simulink model "AttitudeOnly"  (R2024b)
settings: Solver=VariableStepAuto  StartTime=0.0  StopTime=10.0  FixedStep=0.00001  RelTol=1e-3
undefined symbols (not defined in the file): d, DiscIntNeverNeededParam, g, I, k_q, k_t, m, rad, s, Ts_PID_attitude, Ts_PID_position
libraries: simulink_extras x10, simulink x6, aerolibconvert2 x4, aerolibutil x2, shared6dof x1, matrix_library x1, sharedutil x1
settings Model: Creator=User  LastModifiedBy=User

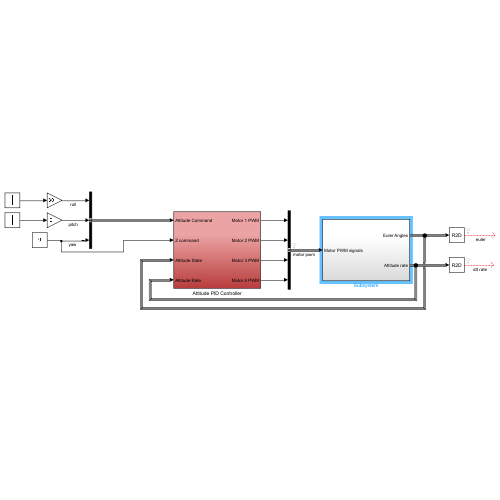
[thumbnail: Simulink's stored preview of the top-level diagram]
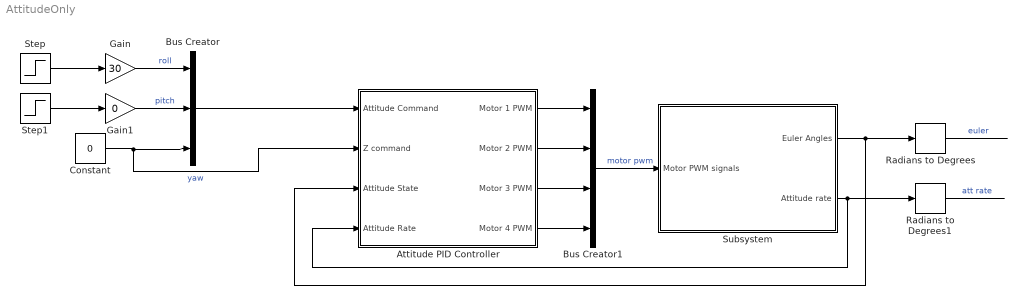
== system AttitudeOnly ==
  Attitude PID Controller : Subsystem
  Bus Creator : BusCreator  Inputs=3
  Bus Creator1 : BusCreator  Inputs=4
  Constant : Constant  Value=0
  Gain : Gain  Gain=30
  Gain1 : Gain  Gain=0
  Radians to Degrees : simulink_extras/Transformations/Radians to Degrees
  Radians to Degrees1 : simulink_extras/Transformations/Radians to Degrees
  Step : Step  Time=2  SampleTime=0
  Step1 : Step  Time=2  SampleTime=0
  Subsystem : Subsystem
  wires:
  Attitude PID Controller/2(Motor 2 PWM) -> Bus Creator1/2
  Attitude PID Controller/1(Motor 1 PWM) -> Bus Creator1/1
  Attitude PID Controller/3(Motor 3 PWM) -> Bus Creator1/3
  Attitude PID Controller/4(Motor 4 PWM) -> Bus Creator1/4
  Bus Creator1/1 -> Subsystem/1(Motor PWM signals)  "motor pwm"
  Bus Creator/1 -> Attitude PID Controller/1(Attitude Command)
  Step1/1 -> Gain1/1
  Constant/1 -> Bus Creator/3, Attitude PID Controller/2(Z command)  "yaw"
  Step/1 -> Gain/1
  Gain/1 -> Bus Creator/1  "roll"
  Gain1/1 -> Bus Creator/2  "pitch"
  Subsystem/1(Euler Angles) -> Radians to Degrees/1, Attitude PID Controller/3(Attitude State)
  Subsystem/2(Attitude rate) -> Radians to Degrees1/1, Attitude PID Controller/4(Attitude Rate)
  Radians to Degrees/1 -> ?  "euler"
  Radians to Degrees1/1 -> ?  "att rate"

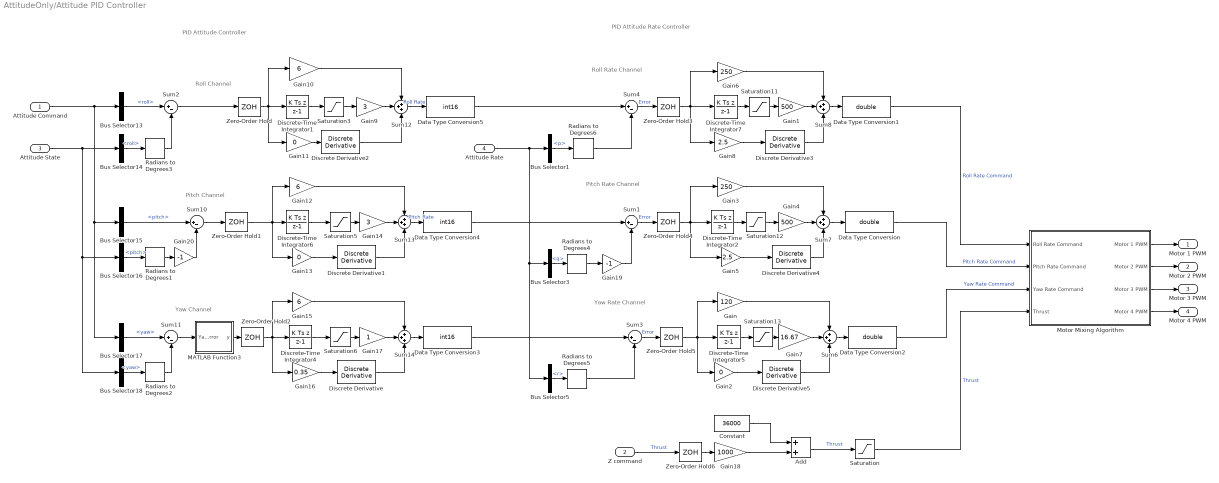
== system AttitudeOnly/Attitude PID Controller ==
  note: Yaw Rate Channel
  note: Pitch Rate Channel
  note: Roll Rate Channel
  note: Yaw Channel
  note: Pitch Channel
  note: PID Attitude Rate Controller
  note: PID Attitude Controller
  note: Roll Channel
  Attitude Command : Inport
  Z command : Inport  Port=2
  Attitude State : Inport  Port=3
  Attitude Rate : Inport  Port=4
  Add : Sum
  Bus Selector1 : BusSelector  OutputSignals=p
  Bus Selector13 : BusSelector  OutputSignals=roll
  Bus Selector14 : BusSelector  OutputSignals=roll
  Bus Selector15 : BusSelector  OutputSignals=pitch
  Bus Selector16 : BusSelector  OutputSignals=pitch
  Bus Selector17 : BusSelector  OutputSignals=yaw
  Bus Selector18 : BusSelector  OutputSignals=yaw
  Bus Selector3 : BusSelector  OutputSignals=q
  Bus Selector5 : BusSelector  OutputSignals=r
  Constant : Constant  Value=36000
  Data Type Conversion : DataTypeConversion  OutDataTypeStr=double  RndMeth=Floor
  Data Type Conversion1 : DataTypeConversion  OutDataTypeStr=double  RndMeth=Floor
  Data Type Conversion2 : DataTypeConversion  OutDataTypeStr=double  RndMeth=Floor
  Data Type Conversion3 : DataTypeConversion  OutDataTypeStr=int16  RndMeth=Floor
  Data Type Conversion4 : DataTypeConversion  OutDataTypeStr=int16  RndMeth=Floor
  Data Type Conversion5 : DataTypeConversion  OutDataTypeStr=int16  RndMeth=Floor
  Discrete Derivative{,1..5} (6 alike) : simulink/Discrete/Discrete Derivative  gainval=1.0  ICPrevScaledInput=0.0  OutMin=[]  OutMax=[]  OutDataType=fixdt(1, 16)  OutScaling=2^-10  DoSatur=off
  Discrete-Time Integrator{1..2,4..7} (6 alike) : DiscreteIntegrator  IntegratorMethod=Integration: Backward Euler  SampleTime=-1  ICPrevOutput=DiscIntNeverNeededParam  ICPrevScaledInput=DiscIntNeverNeededParam
  Gain : Gain  Gain=120
  Gain1 : Gain  Gain=500
  Gain10 : Gain  Gain=6
  Gain11 : Gain  Gain=0
  Gain12 : Gain  Gain=6
  Gain13 : Gain  Gain=0
  Gain14 : Gain  Gain=3
  Gain15 : Gain  Gain=6
  Gain16 : Gain  Gain=0.35
  Gain17 : Gain
  Gain18 : Gain  Gain=1000
  Gain19 : Gain  Gain=-1
  Gain2 : Gain  Gain=0
  Gain20 : Gain  Gain=-1
  Gain3 : Gain  Gain=250
  Gain4 : Gain  Gain=500
  Gain5 : Gain  Gain=2.5
  Gain6 : Gain  Gain=250
  Gain7 : Gain  Gain=16.67
  Gain8 : Gain  Gain=2.5
  Gain9 : Gain  Gain=3
  MATLAB Function3 : MATLAB Function  TreatAsAtomicUnit=on
  Motor Mixing Algorithm : Subsystem
  Radians to Degrees{1..6} (6 alike) : simulink_extras/Transformations/Radians to Degrees
  Saturation : Saturate  UpperLimit=65535  LowerLimit=20000
  Saturation11 : Saturate  UpperLimit=33.3  LowerLimit=-33.3
  Saturation12 : Saturate  UpperLimit=33.3  LowerLimit=-33.3
  Saturation13 : Saturate  UpperLimit=166.7  LowerLimit=-166.7
  Saturation3 : Saturate  UpperLimit=20  LowerLimit=-20
  Saturation5 : Saturate  UpperLimit=20  LowerLimit=-20
  Saturation6 : Saturate  UpperLimit=360  LowerLimit=-360
  Sum{1..4,10..11} (6 alike) : Sum  Inputs=|+-
  Sum{6..8,12..14} (6 alike) : Sum  Inputs=+++
  Zero-Order Hold{,1..5} (6 alike) : ZeroOrderHold  SampleTime=Ts_PID_attitude
  Zero-Order Hold6 : ZeroOrderHold  SampleTime=Ts_PID_position
  Motor 1 PWM : Outport
  Motor 2 PWM : Outport  Port=2
  Motor 3 PWM : Outport  Port=3
  Motor 4 PWM : Outport  Port=4
  wires:
  Constant/1 -> Add/1
  Add/1 -> Saturation/1  "Thrust"
  Bus Selector17/1 -> Sum11/1  "<yaw>"
  Motor Mixing Algorithm/4(Motor 4 PWM) -> Motor 4 PWM/1
  Motor Mixing Algorithm/3(Motor 3 PWM) -> Motor 3 PWM/1
  Motor Mixing Algorithm/2(Motor 2 PWM) -> Motor 2 PWM/1
  Motor Mixing Algorithm/1(Motor 1 PWM) -> Motor 1 PWM/1
  Sum13/1 -> Data Type Conversion4/1  "Pitch Rate"
  Sum12/1 -> Data Type Conversion5/1  "Roll Rate"
  Sum11/1 -> MATLAB Function3/1(YawError)
  Zero-Order Hold2/1 -> Discrete-Time Integrator4/1, Gain16/1, Gain15/1
  Radians to Degrees2/1 -> Sum11/2
  Saturation6/1 -> Gain17/1
  Saturation5/1 -> Gain14/1
  Saturation3/1 -> Gain9/1
  Discrete-Time Integrator4/1 -> Saturation6/1
  Discrete-Time Integrator6/1 -> Saturation5/1
  Discrete-Time Integrator1/1 -> Saturation3/1
  Saturation13/1 -> Gain7/1
  Saturation12/1 -> Gain4/1
  Saturation11/1 -> Gain1/1
  Gain16/1 -> Discrete Derivative/1
  Gain15/1 -> Sum14/1
  Gain12/1 -> Sum13/1
  Sum10/1 -> Zero-Order Hold1/1
  Gain10/1 -> Sum12/1
  Gain11/1 -> Discrete Derivative2/1
  Sum2/1 -> Zero-Order Hold/1
  Bus Selector18/1 -> Radians to Degrees2/1  "<yaw>"
  Bus Selector16/1 -> Radians to Degrees1/1  "<pitch>"
  Bus Selector14/1 -> Radians to Degrees3/1  "<roll>"
  Attitude Command/1 -> Bus Selector17/1, Bus Selector15/1, Bus Selector13/1
  Discrete-Time Integrator5/1 -> Saturation13/1
  Discrete-Time Integrator2/1 -> Saturation12/1
  Discrete-Time Integrator7/1 -> Saturation11/1
  Sum3/1 -> Zero-Order Hold5/1  "Error"
  Gain5/1 -> Discrete Derivative4/1
  Sum6/1 -> Data Type Conversion2/1
  Sum7/1 -> Data Type Conversion/1
  Sum8/1 -> Data Type Conversion1/1
  Sum4/1 -> Zero-Order Hold3/1  "Error"
  Gain6/1 -> Sum8/1
  Sum1/1 -> Zero-Order Hold4/1  "Error"
  Gain3/1 -> Sum7/1
  Gain/1 -> Sum6/1
  Attitude Rate/1 -> Bus Selector5/1, Bus Selector3/1, Bus Selector1/1
  Bus Selector5/1 -> Radians to Degrees5/1  "<r>"
  Bus Selector3/1 -> Radians to Degrees4/1  "<q>"
  Bus Selector1/1 -> Radians to Degrees6/1  "<p>"
  Gain18/1 -> Add/2
  Z command/1 -> Zero-Order Hold6/1  "Thrust"
  Attitude State/1 -> Bus Selector14/1, Bus Selector16/1, Bus Selector18/1
  Saturation/1 -> Motor Mixing Algorithm/4(Thrust)  "Thrust"
  Zero-Order Hold/1 -> Gain10/1, Discrete-Time Integrator1/1, Gain11/1
  Zero-Order Hold1/1 -> Discrete-Time Integrator6/1, Gain12/1, Gain13/1
  MATLAB Function3/1(y) -> Zero-Order Hold2/1
  Zero-Order Hold4/1 -> Discrete-Time Integrator2/1, Gain3/1, Gain5/1
  Zero-Order Hold5/1 -> Discrete-Time Integrator5/1, Gain2/1, Gain/1
  Zero-Order Hold6/1 -> Gain18/1
  Gain2/1 -> Discrete Derivative5/1
  Data Type Conversion4/1 -> Sum1/1
  Data Type Conversion1/1 -> Motor Mixing Algorithm/1(Roll Rate Command)  "Roll Rate Command"
  Data Type Conversion/1 -> Motor Mixing Algorithm/2(Pitch Rate Command)  "Pitch Rate Command"
  Data Type Conversion2/1 -> Motor Mixing Algorithm/3(Yaw Rate Command)  "Yaw Rate Command"
  Gain13/1 -> Discrete Derivative1/1
  Zero-Order Hold3/1 -> Discrete-Time Integrator7/1, Gain6/1, Gain8/1
  Gain8/1 -> Discrete Derivative3/1
  Gain4/1 -> Sum7/2
  Gain9/1 -> Sum12/2
  Gain17/1 -> Sum14/2
  Gain1/1 -> Sum8/2
  Gain14/1 -> Sum13/2
  Gain7/1 -> Sum6/2
  Bus Selector13/1 -> Sum2/1  "<roll>"
  Data Type Conversion5/1 -> Sum4/1
  Bus Selector15/1 -> Sum10/1  "<pitch>"
  Discrete Derivative3/1 -> Sum8/3
  Discrete Derivative4/1 -> Sum7/3
  Discrete Derivative/1 -> Sum14/3
  Discrete Derivative1/1 -> Sum13/3
  Discrete Derivative2/1 -> Sum12/3
  Sum14/1 -> Data Type Conversion3/1
  Data Type Conversion3/1 -> Sum3/1
  Discrete Derivative5/1 -> Sum6/3
  Radians to Degrees3/1 -> Sum2/2
  Radians to Degrees1/1 -> Gain20/1
  Gain20/1 -> Sum10/2
  Gain19/1 -> Sum1/2
  Radians to Degrees6/1 -> Sum4/2
  Radians to Degrees4/1 -> Gain19/1
  Radians to Degrees5/1 -> Sum3/2

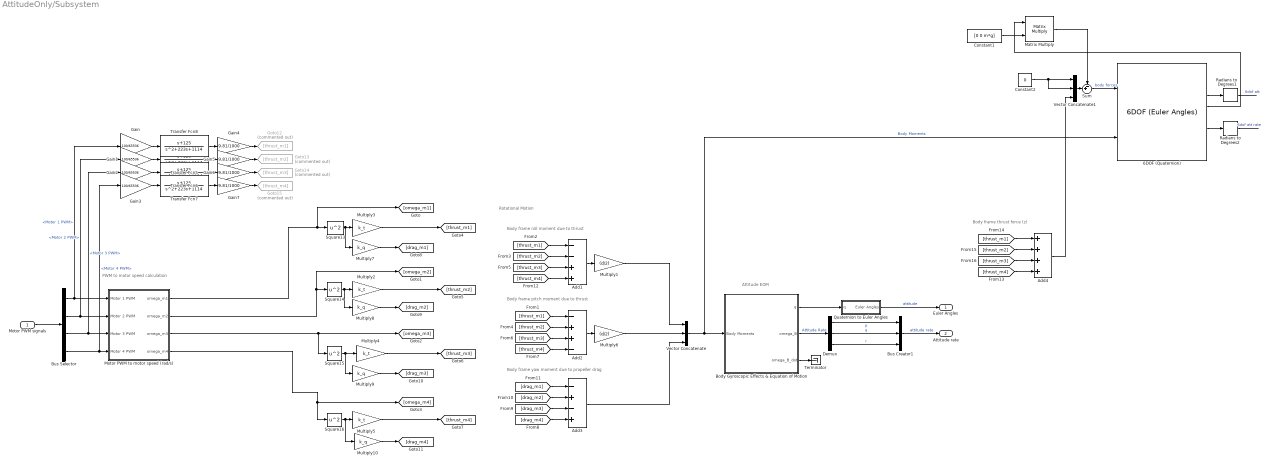
== system AttitudeOnly/Subsystem ==
  note: Body frame pitch moment due to thrust
  note: PWM to motor
      | speed calculation
  note: Rotational Motion
  note: Body frame roll moment due to thrust
  note: Attitude EOM
  note: Body frame yaw moment due to propeller drag
  note: Body frame thrust force (z)
  Motor PWM signals : Inport
  6DOF (Quaternion) : shared6dof/6DOF (Euler Angles)  units=Metric (MKS)  mtype=Fixed  rep=Quaternion  xme_0=[0 0 0.5]  Vm_0=[0 0 0]  eul_0=[0 0 0]  pm_0=[0 0 0]  mass_0=m  mass_e=0.5  mass_f=2.0  inertia=I  inertia_e=eye(3)  inertia_f=2*eye(3)  k_quat=1.0  vre_flag=on  abi_flag=off  aMode=0  xme_statename=''  Vm_statename=''  eul_statename=''  quat_statename=''  pm_statename=''  mass_statename=''
      settings: LibrarySourceBlock=aerolib6dof2/6DOF (Quaternion)
  Add1 : Sum  Inputs=--++
  Add2 : Sum  Inputs=-++-
  Add3 : Sum  Inputs=-+-+
  Add4 : Sum  Inputs=++++
  Body Gyroscopic Effects & Equation of Motion : Subsystem
  Bus Creator1 : BusCreator  Inputs=3
  Bus Selector : BusSelector  OutputSignals=Motor 1 PWM,Motor 2 PWM,Motor 3 PWM,Motor 4 PWM
  Constant1 : Constant  Value=[0 0 m*g]
  Constant2 : Constant  Value=0
  Demux : Demux  Outputs=3
  Gain{,1..3} (4 alike) : Gain  Gain=100/65536
  Gain{4..7} (4 alike) : Gain  Gain=9.81/1000
  Goto12 : Goto  Commented=on  GotoTag=thrust_m1
  Goto13 : Goto  Commented=on  GotoTag=thrust_m2
  Goto14 : Goto  Commented=on  GotoTag=thrust_m3
  Goto15 : Goto  Commented=on  GotoTag=thrust_m4
  Matrix Multiply : Product  Multiplication=Matrix(*)
  Motor PWM to motor speed (rad/s) : Subsystem
  Multiply1 : Gain  Gain=(d/2)
  Multiply{7..10} (4 alike) : Gain  Gain=k_q
  Multiply{2..5} (4 alike) : Gain  Gain=k_t
  Multiply6 : Gain  Gain=(d/2)
  Quaternion to Euler Angles : Subsystem
  Radians to Degrees1 : simulink_extras/Transformations/Radians to Degrees
  Radians to Degrees2 : simulink_extras/Transformations/Radians to Degrees
  Square{13..16} (4 alike) : Math  Operator=square
  Sum : Sum  Inputs=-+|
  Terminator : Terminator
  Transfer Fcn{5..8} (4 alike) : TransferFcn  Numerator=[1 125]  Denominator=[1 223 1114]
  Vector Concatenate : Concatenate  NumInputs=3
  Vector Concatenate1 : Concatenate  NumInputs=3
  Euler Angles : Outport
  Attitude rate : Outport  Port=2
  wires:
  Multiply7/1 -> [drag_m1]
  [thrust_m3] -> Add1/3
  [thrust_m4] -> Add2/4
  Square13/1 -> Multiply3/1, Multiply7/1
  [drag_m4] -> Add3/4
  Body Gyroscopic Effects & Equation of Motion/3(omega_B_dot) -> Terminator/1
  Bus Selector/4 -> Gain3/1, Motor PWM to motor speed (rad/s)/4(Motor 4 PWM)  "<Motor 4 PWM>"
  Multiply4/1 -> [thrust_m3]
  [thrust_m2] -> Add2/2
  Add2/1 -> Multiply6/1
  [thrust_m2] -> Add1/2
  Motor PWM signals/1 -> Bus Selector/1
  Motor PWM to motor speed (rad/s)/3(omega_m3) -> [omega_m3], Square15/1
  Square16/1 -> Multiply10/1, Multiply5/1
  Multiply8/1 -> [drag_m2]
  [drag_m1] -> Add3/1
  [thrust_m1] -> Add2/1
  Multiply1/1 -> Vector Concatenate/1
  Bus Selector/1 -> Gain/1, Motor PWM to motor speed (rad/s)/1(Motor 1 PWM)  "<Motor 1 PWM>"
  Multiply3/1 -> [thrust_m1]
  Multiply10/1 -> [drag_m4]
  Bus Selector/2 -> Gain1/1, Motor PWM to motor speed (rad/s)/2(Motor 2 PWM)  "<Motor 2 PWM>"
  Add3/1 -> Vector Concatenate/3
  Square15/1 -> Multiply9/1, Multiply4/1
  Multiply6/1 -> Vector Concatenate/2
  [thrust_m4] -> Add1/4
  [drag_m3] -> Add3/3
  Motor PWM to motor speed (rad/s)/2(omega_m2) -> [omega_m2], Square14/1
  Add1/1 -> Multiply1/1
  [drag_m2] -> Add3/2
  Multiply2/1 -> [thrust_m2]
  Motor PWM to motor speed (rad/s)/1(omega_m1) -> [omega_m1], Square13/1
  Bus Selector/3 -> Gain2/1, Motor PWM to motor speed (rad/s)/3(Motor 3 PWM)  "<Motor 3 PWM>"
  [thrust_m3] -> Add2/3
  Multiply9/1 -> [drag_m3]
  [thrust_m1] -> Add1/1
  Motor PWM to motor speed (rad/s)/4(omega_m4) -> [omega_m4], Square16/1
  Multiply5/1 -> [thrust_m4]
  Square14/1 -> Multiply8/1, Multiply2/1
  Body Gyroscopic Effects & Equation of Motion/1(q) -> Quaternion to Euler Angles/1(q)
  Quaternion to Euler Angles/1(Euler Angles) -> Euler Angles/1  "attitude"
  Demux/3 -> Bus Creator1/3  "r"
  Bus Creator1/1 -> Attitude rate/1  "attitude rate"
  Body Gyroscopic Effects & Equation of Motion/2(omega_B) -> Demux/1  "Attitude Rate"
  Demux/2 -> Bus Creator1/2  "q"
  Demux/1 -> Bus Creator1/1  "p"
  Transfer Fcn8/1 -> Gain4/1
  Gain/1 -> Transfer Fcn8/1
  Gain1/1 -> Transfer Fcn5/1
  Transfer Fcn5/1 -> Gain5/1
  Gain2/1 -> Transfer Fcn6/1
  Transfer Fcn6/1 -> Gain6/1
  Gain3/1 -> Transfer Fcn7/1
  Transfer Fcn7/1 -> Gain7/1
  Matrix Multiply/1 -> Sum/1
  6DOF (Quaternion)/4 -> Matrix Multiply/1
  Add4/1 -> Vector Concatenate1/3
  Vector Concatenate1/1 -> Sum/2
  Constant1/1 -> Matrix Multiply/2
  Constant2/1 -> Vector Concatenate1/2, Vector Concatenate1/1
  Sum/1 -> 6DOF (Quaternion)/1  "body forces"
  Vector Concatenate/1 -> 6DOF (Quaternion)/2, Body Gyroscopic Effects & Equation of Motion/1(Body Moments)  "Body Moments"
  6DOF (Quaternion)/3 -> Radians to Degrees1/1
  [thrust_m3] -> Add4/3
  [thrust_m2] -> Add4/2
  [thrust_m4] -> Add4/4
  [thrust_m1] -> Add4/1
  Radians to Degrees1/1 -> ?  "6dof att"
  6DOF (Quaternion)/6 -> Radians to Degrees2/1
  Radians to Degrees2/1 -> ?  "6dof att rate"
  Gain4/1 -> Goto12/1
  Gain5/1 -> Goto13/1
  Gain6/1 -> Goto14/1
  Gain7/1 -> Goto15/1

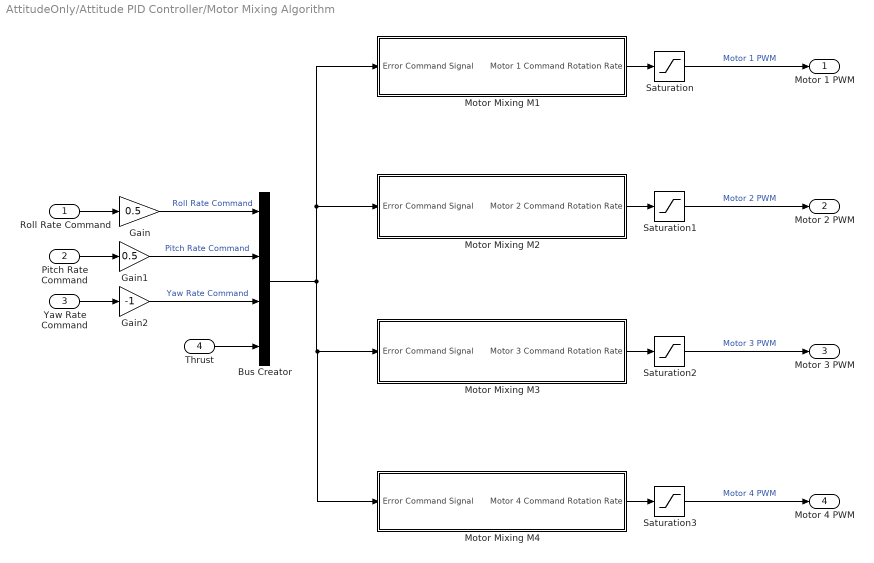
== system AttitudeOnly/Attitude PID Controller/Motor Mixing Algorithm ==
  Roll Rate Command : Inport
  Pitch Rate Command : Inport  Port=2
  Yaw Rate Command : Inport  Port=3
  Thrust : Inport  Port=4
  Bus Creator : BusCreator  Inputs=4
  Gain : Gain  Gain=0.5
  Gain1 : Gain  Gain=0.5
  Gain2 : Gain  Gain=-1
  Motor Mixing M1 : Subsystem
  Motor Mixing M2 : Subsystem
  Motor Mixing M3 : Subsystem
  Motor Mixing M4 : Subsystem
  Saturation : Saturate  UpperLimit=65536  LowerLimit=-0  LinearizeAsGain=off  ZeroCross=off
  Saturation1 : Saturate  UpperLimit=65536  LowerLimit=-0  LinearizeAsGain=off  ZeroCross=off
  Saturation2 : Saturate  UpperLimit=65536  LowerLimit=0.  LinearizeAsGain=off  ZeroCross=off
  Saturation3 : Saturate  UpperLimit=65536  LowerLimit=0  LinearizeAsGain=off  ZeroCross=off
  Motor 1 PWM : Outport
  Motor 2 PWM : Outport  Port=2
  Motor 3 PWM : Outport  Port=3
  Motor 4 PWM : Outport  Port=4
  wires:
  Saturation3/1 -> Motor 4 PWM/1  "Motor 4 PWM"
  Saturation2/1 -> Motor 3 PWM/1  "Motor 3 PWM"
  Saturation1/1 -> Motor 2 PWM/1  "Motor 2 PWM"
  Saturation/1 -> Motor 1 PWM/1  "Motor 1 PWM"
  Bus Creator/1 -> Motor Mixing M3/1(Error Command Signal), Motor Mixing M4/1(Error Command Signal), Motor Mixing M1/1(Error Command Signal), Motor Mixing M2/1(Error Command Signal)
  Thrust/1 -> Bus Creator/4
  Motor Mixing M1/1(Motor 1 Command Rotation Rate) -> Saturation/1
  Motor Mixing M2/1(Motor 2 Command Rotation Rate) -> Saturation1/1
  Motor Mixing M4/1(Motor 4 Command Rotation Rate) -> Saturation3/1
  Motor Mixing M3/1(Motor 3 Command Rotation Rate) -> Saturation2/1
  Gain/1 -> Bus Creator/1  "Roll Rate Command"
  Gain1/1 -> Bus Creator/2  "Pitch Rate Command"
  Pitch Rate Command/1 -> Gain1/1
  Roll Rate Command/1 -> Gain/1
  Yaw Rate Command/1 -> Gain2/1
  Gain2/1 -> Bus Creator/3  "Yaw Rate Command"

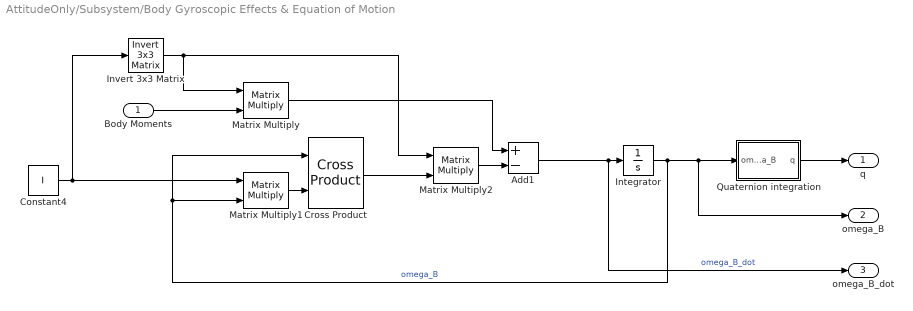
== system AttitudeOnly/Subsystem/Body Gyroscopic Effects & Equation of Motion ==
  Body Moments : Inport
  Add1 : Sum  Inputs=+-
  Constant4 : Constant  Value=I
  Cross Product : matrix_library/Cross Product
  Integrator : Integrator
  Invert 3x3 Matrix : aerolibutil/Invert  3x3 Matrix
  Matrix Multiply : Product  Multiplication=Matrix(*)
  Matrix Multiply1 : Product  Multiplication=Matrix(*)
  Matrix Multiply2 : Product  Multiplication=Matrix(*)
  Quaternion integration : Subsystem
  q : Outport
  omega_B : Outport  Port=2
  omega_B_dot : Outport  Port=3
  wires:
  Quaternion integration/1(q) -> q/1
  Body Moments/1 -> Matrix Multiply/2
  Invert 3x3 Matrix/1 -> Matrix Multiply/1, Matrix Multiply2/1
  Integrator/1 -> Matrix Multiply1/2, Cross Product/1, Quaternion integration/1(omega_B), omega_B/1  "omega_B"
  Cross Product/1 -> Matrix Multiply2/2
  Matrix Multiply/1 -> Add1/1
  Matrix Multiply1/1 -> Cross Product/2
  Matrix Multiply2/1 -> Add1/2
  Add1/1 -> omega_B_dot/1, Integrator/1  "omega_B_dot"
  Constant4/1 -> Matrix Multiply1/1, Invert 3x3 Matrix/1

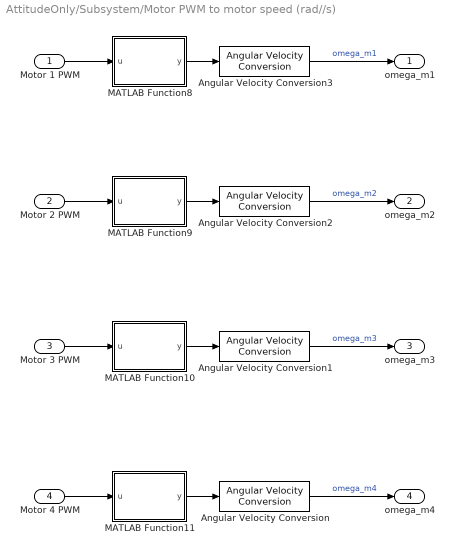
== system AttitudeOnly/Subsystem/Motor PWM to motor speed (rad//s) ==
  Motor 1 PWM : Inport
  Motor 2 PWM : Inport  Port=2
  Motor 3 PWM : Inport  Port=3
  Motor 4 PWM : Inport  Port=4
  Angular Velocity Conversion{,1..3} (4 alike) : aerolibconvert2/Angular Velocity Conversion  IU=rpm  OU=rad/s
  MATLAB Function10 : MATLAB Function  TreatAsAtomicUnit=on
  MATLAB Function11 : MATLAB Function  TreatAsAtomicUnit=on
  MATLAB Function8 : MATLAB Function  TreatAsAtomicUnit=on
  MATLAB Function9 : MATLAB Function  TreatAsAtomicUnit=on
  omega_m1 : Outport
  omega_m2 : Outport  Port=2
  omega_m3 : Outport  Port=3
  omega_m4 : Outport  Port=4
  wires:
  Motor 4 PWM/1 -> MATLAB Function11/1(u)
  Motor 3 PWM/1 -> MATLAB Function10/1(u)
  Motor 2 PWM/1 -> MATLAB Function9/1(u)
  Motor 1 PWM/1 -> MATLAB Function8/1(u)
  MATLAB Function10/1(y) -> Angular Velocity Conversion1/1
  Angular Velocity Conversion3/1 -> omega_m1/1  "omega_m1"
  MATLAB Function8/1(y) -> Angular Velocity Conversion3/1
  Angular Velocity Conversion2/1 -> omega_m2/1  "omega_m2"
  MATLAB Function11/1(y) -> Angular Velocity Conversion/1
  Angular Velocity Conversion/1 -> omega_m4/1  "omega_m4"
  Angular Velocity Conversion1/1 -> omega_m3/1  "omega_m3"
  MATLAB Function9/1(y) -> Angular Velocity Conversion2/1

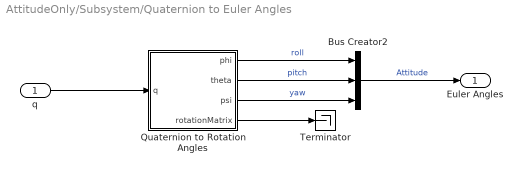
== system AttitudeOnly/Subsystem/Quaternion to Euler Angles ==
  q : Inport
  Bus Creator2 : BusCreator  Inputs=3
  Quaternion to Rotation Angles : MATLAB Function  TreatAsAtomicUnit=on
  Terminator : Terminator
  Euler Angles : Outport
  wires:
  Quaternion to Rotation Angles/4(rotationMatrix) -> Terminator/1
  q/1 -> Quaternion to Rotation Angles/1(q)
  Quaternion to Rotation Angles/2(theta) -> Bus Creator2/2  "pitch"
  Quaternion to Rotation Angles/3(psi) -> Bus Creator2/3  "yaw"
  Quaternion to Rotation Angles/1(phi) -> Bus Creator2/1  "roll"
  Bus Creator2/1 -> Euler Angles/1  "Attitude"

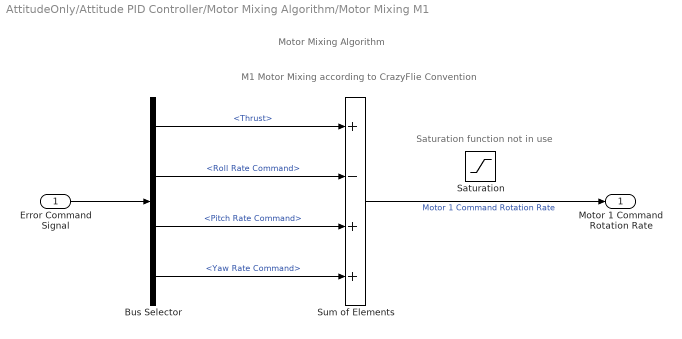
== system AttitudeOnly/Attitude PID Controller/Motor Mixing Algorithm/Motor Mixing M1 ==
  note: Saturation function not in use
  note: M1 Motor Mixing according to CrazyFlie Convention
  note: Motor Mixing Algorithm
  Error Command Signal : Inport
  Bus Selector : BusSelector  OutputSignals=Thrust,Roll Rate Command,Pitch Rate Command,Yaw Rate Command
  Saturation : Saturate
  Sum of Elements : Sum  Inputs=+-++
  Motor 1 Command Rotation Rate : Outport
  wires:
  Bus Selector/1 -> Sum of Elements/1  "<Thrust>"
  Bus Selector/2 -> Sum of Elements/2  "<Roll Rate Command>"
  Bus Selector/4 -> Sum of Elements/4  "<Yaw Rate Command>"
  Bus Selector/3 -> Sum of Elements/3  "<Pitch Rate Command>"
  Sum of Elements/1 -> Motor 1 Command Rotation Rate/1  "Motor 1 Command Rotation Rate"
  Error Command Signal/1 -> Bus Selector/1

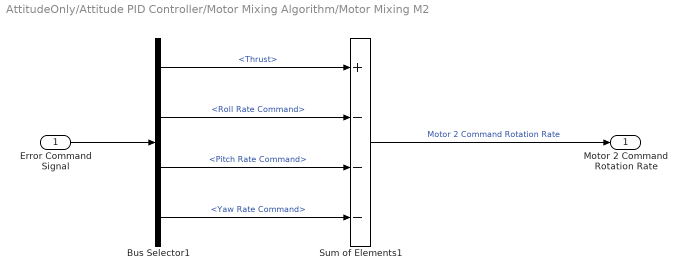
== system AttitudeOnly/Attitude PID Controller/Motor Mixing Algorithm/Motor Mixing M2 ==
  Error Command Signal : Inport
  Bus Selector1 : BusSelector  OutputSignals=Thrust,Roll Rate Command,Pitch Rate Command,Yaw Rate Command
  Sum of Elements1 : Sum  Inputs=+---
  Motor 2 Command Rotation Rate : Outport
  wires:
  Sum of Elements1/1 -> Motor 2 Command Rotation Rate/1  "Motor 2 Command Rotation Rate"
  Bus Selector1/2 -> Sum of Elements1/2  "<Roll Rate Command>"
  Bus Selector1/1 -> Sum of Elements1/1  "<Thrust>"
  Bus Selector1/3 -> Sum of Elements1/3  "<Pitch Rate Command>"
  Error Command Signal/1 -> Bus Selector1/1
  Bus Selector1/4 -> Sum of Elements1/4  "<Yaw Rate Command>"

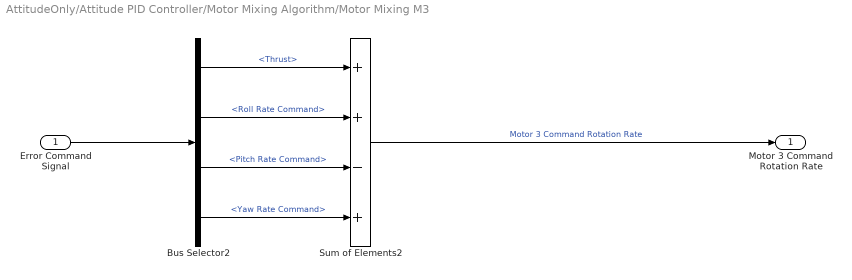
== system AttitudeOnly/Attitude PID Controller/Motor Mixing Algorithm/Motor Mixing M3 ==
  Error Command Signal : Inport
  Bus Selector2 : BusSelector  OutputSignals=Thrust,Roll Rate Command,Pitch Rate Command,Yaw Rate Command
  Sum of Elements2 : Sum  Inputs=++-+
  Motor 3 Command Rotation Rate : Outport
  wires:
  Sum of Elements2/1 -> Motor 3 Command Rotation Rate/1  "Motor 3 Command Rotation Rate"
  Bus Selector2/3 -> Sum of Elements2/3  "<Pitch Rate Command>"
  Bus Selector2/4 -> Sum of Elements2/4  "<Yaw Rate Command>"
  Error Command Signal/1 -> Bus Selector2/1
  Bus Selector2/1 -> Sum of Elements2/1  "<Thrust>"
  Bus Selector2/2 -> Sum of Elements2/2  "<Roll Rate Command>"

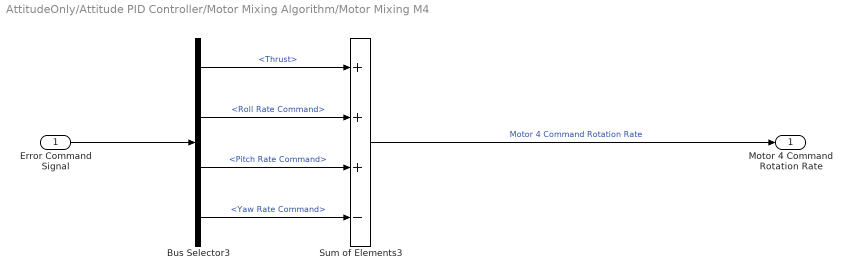
== system AttitudeOnly/Attitude PID Controller/Motor Mixing Algorithm/Motor Mixing M4 ==
  Error Command Signal : Inport
  Bus Selector3 : BusSelector  OutputSignals=Thrust,Roll Rate Command,Pitch Rate Command,Yaw Rate Command
  Sum of Elements3 : Sum  Inputs=+++-
  Motor 4 Command Rotation Rate : Outport
  wires:
  Error Command Signal/1 -> Bus Selector3/1
  Bus Selector3/3 -> Sum of Elements3/3  "<Pitch Rate Command>"
  Bus Selector3/1 -> Sum of Elements3/1  "<Thrust>"
  Sum of Elements3/1 -> Motor 4 Command Rotation Rate/1  "Motor 4 Command Rotation Rate"
  Bus Selector3/2 -> Sum of Elements3/2  "<Roll Rate Command>"
  Bus Selector3/4 -> Sum of Elements3/4  "<Yaw Rate Command>"

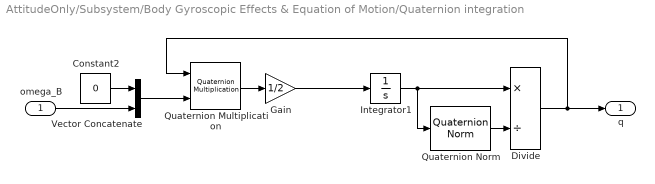
== system AttitudeOnly/Subsystem/Body Gyroscopic Effects & Equation of Motion/Quaternion integration ==
  omega_B : Inport
  Constant2 : Constant  Value=0
  Divide : Product  Inputs=*/
  Gain : Gain  Gain=1/2
  Integrator1 : Integrator  InitialCondition=[1 0 0 0]'
  Quaternion Multiplication : aerolibutil/Quaternion Multiplication
  Quaternion Norm : sharedutil/Quaternion Norm  aMode=aMode
      settings: LibrarySourceBlock=|
      | aerolibutil/Quaternion
      | Norm
  Vector Concatenate : Concatenate
  q : Outport
  wires:
  omega_B/1 -> Vector Concatenate/2
  Quaternion Norm/1 -> Divide/2
  Gain/1 -> Integrator1/1
  Vector Concatenate/1 -> Quaternion Multiplication/2
  Quaternion Multiplication/1 -> Gain/1
  Constant2/1 -> Vector Concatenate/1
  Integrator1/1 -> Divide/1, Quaternion Norm/1
  Divide/1 -> q/1, Quaternion Multiplication/1

== matlab function AttitudeOnly/Subsystem/Motor PWM to motor speed (rad//s)/MATLAB Function10 ==
  data: u input; y output
function y = PWMtoRPM(u)

y = u*0.2685+4070.3;

== matlab function AttitudeOnly/Subsystem/Motor PWM to motor speed (rad//s)/MATLAB Function11 ==
  data: u input; y output
function y = PWMtoRPM(u)

y = u*0.2685+4070.3;

== matlab function AttitudeOnly/Subsystem/Motor PWM to motor speed (rad//s)/MATLAB Function8 ==
  data: u input; y output
function y = PWMtoRPM(u)

y = u*0.2685+4070.3;

== matlab function AttitudeOnly/Subsystem/Motor PWM to motor speed (rad//s)/MATLAB Function9 ==
  data: u input; y output
function y = PWMtoRPM(u)

y = u*0.2685+4070.3;

== matlab function AttitudeOnly/Subsystem/Quaternion to Euler Angles/Quaternion to Rotation Angles ==
  data: q input; phi output; theta output; psi output; rotationMatrix output
function [phi, theta, psi, rotationMatrix] = fcn(q)

q_0 = q(1);
q_x = q(2);
q_y = q(3);
q_z = q(4);

R_11 = 2*(q_0^2 + q_x^2) - 1;
R_12 = 2*(q_x*q_y - q_0*q_z);
R_13 = 2*(q_x*q_z + q_0*q_y);

R_21 = 2*(q_x*q_y + q_0*q_z);
R_22 = 2*(q_0^2 + q_y^2) - 1;
R_23 = 2*(q_y*q_z - q_0*q_x);

R_31 = 2*(q_x*q_z - q_0*q_y);
R_32 = 2*(q_y*q_z + q_0*q_x);
R_33 = 2*(q_0^2 + q_z^2) - 1;

phi = atan2(R_32, R_33);
theta = -atan2(R_31, sqrt(1 - (R_31^2)));
psi = atan2(R_21, R_11);

rotationMatrix = [R_11 R_12 R_13;...
        R_21 R_22 R_23;...
        R_31 R_32 R_33];

== matlab function AttitudeOnly/Attitude PID Controller/MATLAB Function3 ==
  data: YawError input; y output
function y = fcn(YawError)
YawError1=YawError;
if YawError>180
    YawError1=YawError-360;
end 
if YawError<-180
    YawError1=YawError+360;
end

y = YawError1;
